simulink model "testBCIRobot3c"  (Simulink 10.0)
settings: Solver=FixedStepDiscrete  StartTime=0.0  StopTime=inf  FixedStep=0.002  MaxStep=0.02  RelTol=1e-3  AbsTol=1e-6
settings Model: Creator=fwornle  LastModifiedBy=bhisma  SimulationMode=external  ExtModeTrigDuration=5000  ExtModeLogAll=off
settings ConfigSet: Description=rtmc9s12target_R2009b
settings SolverCC: AutoScaleAbsTol=off
settings DataIOCC: SignalLoggingSaveFormat=ModelDataLogs  SaveOutput=off  SaveTime=off  SignalLoggingName=sigsOut
settings OptimizationCC: BlockReduction=off  BooleanDataType=off  ExpressionDepthLimit=2147483647  InitFltsAndDblsToZero=on  LifeSpan=1  EfficientTunableParamExpr=on
settings DebuggingCC: SaveWithParameterizedLinksMsg=none  SignalResolutionControl=TryResolveAllWithWarning  MultiTaskDSMMsg=warning  MultiTaskCondExecSysMsg=none  FcnCallInpInsideContextMsg=warning  StateNameClashWarn=warning
settings HardwareCC: ProdBitPerInt=16  ProdBitPerPointer=16  ProdBitPerSizeT=16  ProdBitPerPtrDiffT=16  ProdEndianess=BigEndian  ProdWordSize=16  ProdHWDeviceType=Motorola HC12
settings SFSimCC: MATLABDynamicMemAlloc=off
settings RTWCC: SystemTargetFile=mc9s12.tlc  GenerateMakefile=off  TemplateMakefile=mc9s12.tmf
settings CodeAppCC: IgnoreCustomStorageClasses=off  CustomSymbolStrType=$N$R$M  InternalIdentifier=Classic
settings STFCustomTargetCC: TargetFcnLib=ansi_tfl_tmw.mat  ModelReferenceCompliant=off  IncludeMdlTerminateFcn=off  ERTCustomFileBanners=on  SupportNonInlinedSFcns=off  RemoveResetFunc=on  MATLABClassNameForMDSCustomization=Simulink.SoftwareTarget.ERTCustomization  CPPClassGenCompliant=on  SystemTargetFile=mc9s12.tlc
settings ERTTargetCC: TargetFcnLib=ansi_tfl_tmw.mat  MultiwordLength=2048  ModelReferenceCompliant=off  ParMdlRefBuildCompliant=off  CompOptLevelCompliant=off  ConcurrentExecutionCompliant=off  IncludeMdlTerminateFcn=off  CombineOutputUpdateFcns=off  SupportContinuousTime=on  ModelStepFunctionPrototypeControlCompliant=off  GRTInterface=on  UseToolchainInfoCompliant=off  ExtMode=on  ExtModeMexFile=ext_serial_mc9s12_comm  ExtModeMexArgs=1,2,115200  ERTCustomFileTemplate=mc9s12_file_process.tlc  ConvertIfToSwitch=off  SuppressUnreachableDefaultCases=off
settings CustomProperty: DataType=RTWOptions_EnumType_C__Users_fw__SVN_rtmc9s12-target_trunk_rtmc9s12_CW_R2009b_bin_mc9s12_1mc9s12_TargetBoard  Value=MiniDragonPlus-RevE
settings EnumStrPairs: String=Dragon12
settings ConfigComp: CovExternalEMLEnable=off

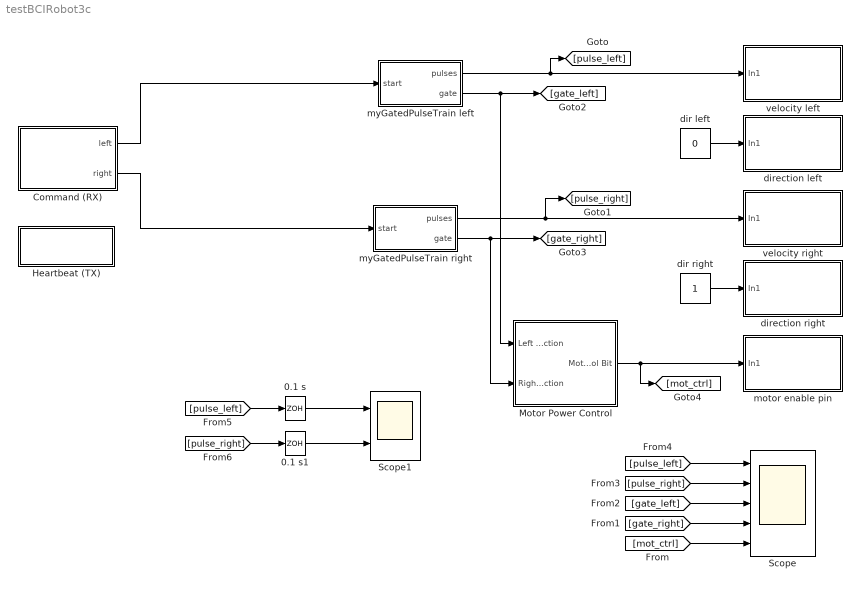
== system testBCIRobot3c ==
  0.1 s : ZeroOrderHold  SampleTime=0.1
  0.1 s1 : ZeroOrderHold  SampleTime=0.1
  Command (RX) : Subsystem
  Heartbeat (TX) : Subsystem  mask{Tbeat=3}
      mask prompts: Tbeat "Period of heartbeat signal (seconds)"
      mask Display: disp(['Tbeat = ' num2str(Tbeat) ' s'])
  Motor Power Control : Subsystem
  Scope : Scope  NumInputPorts=5
  Scope1 : Scope  NumInputPorts=2
  dir left : Constant  Value=0
  dir right : Constant
  direction left : Subsystem  Tag=mcTarget_digOut  mask{port=Port A, pin=5, sampletime=0.002, Von=0.5, Voff=0.5}
      mask prompts: port "Port (see hardware manuals for valid options)"; pin "Pin (see hardware manuals for valid options)"; sampletime "Sample time"; Von "On-threshold (Von)"; Voff "Off-threshold (Voff)"
      mask init:
      | [portstr, pinstr, pins] = mbc_digitaloutput(port, pin, sampletime, Von, Voff);
      mask Help: web('digOut_sfcn_9S12.html');
      mask TypeOptions port: Port A | Port B | Port H | Port J | Port M | Port P | Port S | Port T
      mask Display: fprintf('%s\nPins: %s', portstr, pinstr)
  direction right : Subsystem  Tag=mcTarget_digOut  mask{port=Port A, pin=7, sampletime=0.002, Von=0.5, Voff=0.5}
      mask prompts: port "Port (see hardware manuals for valid options)"; pin "Pin (see hardware manuals for valid options)"; sampletime "Sample time"; Von "On-threshold (Von)"; Voff "Off-threshold (Voff)"
      mask init:
      | [portstr, pinstr, pins] = mbc_digitaloutput(port, pin, sampletime, Von, Voff);
      mask Help: web('digOut_sfcn_9S12.html');
      mask TypeOptions port: Port A | Port B | Port H | Port J | Port M | Port P | Port S | Port T
      mask Display: fprintf('%s\nPins: %s', portstr, pinstr)
  motor enable pin : Subsystem  Tag=mcTarget_digOut  mask{port=Port T, pin=7, sampletime=0.002, Von=0.5, Voff=0.5}
      mask prompts: port "Port (see hardware manuals for valid options)"; pin "Pin (see hardware manuals for valid options)"; sampletime "Sample time"; Von "On-threshold (Von)"; Voff "Off-threshold (Voff)"
      mask init:
      | [portstr, pinstr, pins] = mbc_digitaloutput(port, pin, sampletime, Von, Voff);
      mask Help: web('digOut_sfcn_9S12.html');
      mask TypeOptions port: Port A | Port B | Port H | Port J | Port M | Port P | Port S | Port T
      mask Display: fprintf('%s\nPins: %s', portstr, pinstr)
  myGatedPulseTrain left : Subsystem  mask{Tcount=0.02, Nsamp=30}
      mask prompts: Tcount "Sample time"; Nsamp "Number of samples"
      mask init:
      | % each period has an on-phase and an off-phase
      | Ncount = 2*Nsamp;
  myGatedPulseTrain right : Subsystem  mask{Tcount=0.02, Nsamp=30}
      mask prompts: Tcount "Sample time"; Nsamp "Number of samples"
      mask init:
      | % each period has an on-phase and an off-phase
      | Ncount = 2*Nsamp;
  velocity left : Subsystem  Tag=mcTarget_digOut  mask{port=Port A, pin=4, sampletime=0.002, Von=0.5, Voff=0.5}
      mask prompts: port "Port (see hardware manuals for valid options)"; pin "Pin (see hardware manuals for valid options)"; sampletime "Sample time"; Von "On-threshold (Von)"; Voff "Off-threshold (Voff)"
      mask init:
      | [portstr, pinstr, pins] = mbc_digitaloutput(port, pin, sampletime, Von, Voff);
      mask Help: web('digOut_sfcn_9S12.html');
      mask TypeOptions port: Port A | Port B | Port H | Port J | Port M | Port P | Port S | Port T
      mask Display: fprintf('%s\nPins: %s', portstr, pinstr)
  velocity right : Subsystem  Tag=mcTarget_digOut  mask{port=Port A, pin=6, sampletime=0.002, Von=0.5, Voff=0.5}
      mask prompts: port "Port (see hardware manuals for valid options)"; pin "Pin (see hardware manuals for valid options)"; sampletime "Sample time"; Von "On-threshold (Von)"; Voff "Off-threshold (Voff)"
      mask init:
      | [portstr, pinstr, pins] = mbc_digitaloutput(port, pin, sampletime, Von, Voff);
      mask Help: web('digOut_sfcn_9S12.html');
      mask TypeOptions port: Port A | Port B | Port H | Port J | Port M | Port P | Port S | Port T
      mask Display: fprintf('%s\nPins: %s', portstr, pinstr)
  wires:
  Motor Power Control/1(Motor Control Bit) -> [mot_ctrl], motor enable pin/1(In1)
  myGatedPulseTrain left/2(gate) -> Motor Power Control/1(Left Motor Instruction), [gate_left]
  myGatedPulseTrain right/2(gate) -> Motor Power Control/2(Right Motor  Instruction), [gate_right]
  myGatedPulseTrain left/1(pulses) -> [pulse_left], velocity left/1(In1)
  myGatedPulseTrain right/1(pulses) -> [pulse_right], velocity right/1(In1)
  dir left/1 -> direction left/1(In1)
  dir right/1 -> direction right/1(In1)
  Command (RX)/2(right) -> myGatedPulseTrain right/1(start)
  [mot_ctrl] -> Scope/5
  [pulse_left] -> Scope/1
  [pulse_right] -> Scope/2
  [gate_left] -> Scope/3
  [gate_right] -> Scope/4
  Command (RX)/1(left) -> myGatedPulseTrain left/1(start)
  [pulse_left] -> 0.1 s/1
  [pulse_right] -> 0.1 s1/1
  0.1 s/1 -> Scope1/1
  0.1 s1/1 -> Scope1/2

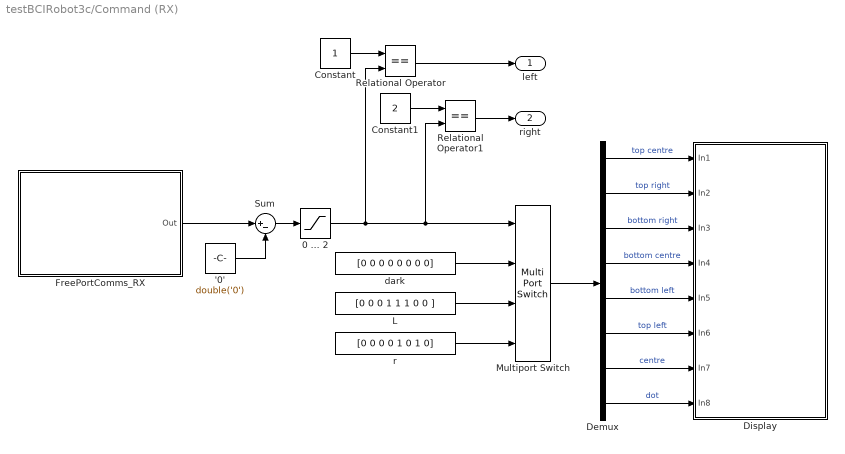
== system testBCIRobot3c/Command (RX) ==
  '0' : Constant  Value=double('0')
  0 ... 2 : Saturate  UpperLimit=2  LowerLimit=0
  Constant : Constant
  Constant1 : Constant  Value=2
  Demux : Demux  Outputs=8
  Display : Subsystem  Tag=mcTarget_digOut  mask{port=Port H, pin=0:7, sampletime=0.1, Von=0.5, Voff=0.5}
      mask prompts: port "Port (see hardware manuals for valid options)"; pin "Pin (see hardware manuals for valid options)"; sampletime "Sample time"; Von "On-threshold (Von)"; Voff "Off-threshold (Voff)"
      mask init:
      | [portstr, pinstr, pins] = mbc_digitaloutput(port, pin, sampletime, Von, Voff);
      mask Help: web('digOut_sfcn_9S12.html');
      mask TypeOptions port: Port A | Port B | Port H | Port J | Port M | Port P | Port S | Port T
      mask Display: fprintf('%s\nPins: %s', portstr, pinstr)
  FreePortComms_RX : Subsystem  Tag=mcTarget_freePortCommsRX  mask{sampletime=0.1, port=SCI0, baudrate=115200, channel=0, buf_size=1, data_type=UINT8, format=on, outformat=on}
      mask prompts: sampletime "Sample time"; port "Communication port"; channel "Channel number"; buf_size "Number of elements"; data_type "Data Type"; format "Block receives raw data"; outformat "Block output is double"
      mask init:
      | [buf_sizestr, portNamestr, baudratestr, channelstr, data_type_str, sampletime_str] = mbc_freeportrxd(sampletime, port, baudrate, channel, buf_size, data_type, format, outformat);
      mask Help: web('freePortComms_rxd.html');
      mask TypeOptions port: SCI0 | SCI1 | COM1 | COM2 | COM3 | COM4
      mask TypeOptions baudrate: 300 | 600 | 1200 | 2400 | 4800 | 9600 | 19200 | 38400 | 57600 | 115200
      mask TypeOptions data_type: SINGLE | INT8 | UINT8 | INT16 | UINT16 | INT32 | UINT32 | BOOLEAN
      mask Display: fprintf('Receive %s element(s)\nComm port: %s\nBaudrate: %s bps\nChannel: %s\nData type: %s\n Sample rate: %s', buf_sizestr, portNamestr, baudratestr, channelstr, data_type_str, sampletime_str)
  L : Constant  Value=[0 0 0 1 1 1 0 0 ]  OutDataTypeStr=double
  Multiport Switch : MultiPortSwitch  DataPortOrder=Zero-based contiguous  zeroidx=on  SaturateOnIntegerOverflow=on
  Relational Operator : RelationalOperator  Operator===  OutDataTypeStr=uint(8)  RndMeth=Nearest
  Relational Operator1 : RelationalOperator  Operator===  OutDataTypeStr=uint(8)  RndMeth=Nearest
  Sum : Sum  Inputs=|+-  SaturateOnIntegerOverflow=on
  dark : Constant  Value=[0 0 0 0 0 0 0 0]  OutDataTypeStr=double
  r : Constant  Value=[0 0 0 0 1 0 1 0]  OutDataTypeStr=double
  left : Outport
  right : Outport  Port=2
  wires:
  dark/1 -> Multiport Switch/2
  L/1 -> Multiport Switch/3
  r/1 -> Multiport Switch/4
  Constant/1 -> Relational Operator/1
  Relational Operator/1 -> left/1
  Constant1/1 -> Relational Operator1/1
  Relational Operator1/1 -> right/1
  Sum/1 -> 0 ... 2/1
  '0'/1 -> Sum/2
  FreePortComms_RX/1(Out) -> Sum/1
  Demux/1 -> Display/1(In1)  "top centre"
  Demux/2 -> Display/2(In2)  "top right"
  Demux/3 -> Display/3(In3)  "bottom right"
  Demux/4 -> Display/4(In4)  "bottom centre"
  Demux/5 -> Display/5(In5)  "bottom left"
  Demux/6 -> Display/6(In6)  "top left"
  Demux/7 -> Display/7(In7)  "centre"
  Demux/8 -> Display/8(In8)  "dot"
  Multiport Switch/1 -> Demux/1
  0 ... 2/1 -> Multiport Switch/1, Relational Operator1/2, Relational Operator/2

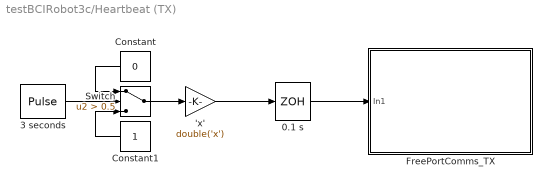
== system testBCIRobot3c/Heartbeat (TX) ==
  'x' : Gain  Gain=double('x')  SaturateOnIntegerOverflow=on  OutDataTypeStr=Inherit: Same as input  ParamDataTypeStr=Inherit: Same as input
  0.1 s : ZeroOrderHold  SampleTime=0.1
  3 seconds : DiscretePulseGenerator  PulseType=Time based  Period=3  PulseWidth=0.2
  Constant : Constant  Value=0
  Constant1 : Constant
  FreePortComms_TX : Subsystem  Tag=mcTarget_freePortCommsTX  mask{sampletime=0.1, port=SCI1, baudrate=115200, channel=0, buf_size=1, data_type=UINT8, format=on}
      mask prompts: sampletime "Sample time"; port "Communication port"; channel "Channel number"; buf_size "Number of elements"; data_type "Data Type"; format "Block sends raw data"
      mask init:
      | [buf_sizestr, portNamestr, baudratestr, channelstr, data_type_str, sampletime_str] = mbc_freeporttxd(sampletime, port, baudrate, channel, buf_size, data_type, format);
      mask Help: web('freePortComms_txd.html');
      mask TypeOptions port: SCI0 | SCI1 | COM1 | COM2 | COM3 | COM4
      mask TypeOptions baudrate: 300 | 600 | 1200 | 2400 | 4800 | 9600 | 19200 | 38400 | 57600 | 115200
      mask TypeOptions data_type: SINGLE | INT8 | UINT8 | INT16 | UINT16 | INT32 | UINT32 | BOOLEAN
      mask Display: fprintf('Transmit %s element(s)\nComm port: %s\nBaudrate: %s bps\nChannel: %s\nData type: %s\n Sample rate: %s', buf_sizestr, portNamestr, baudratestr, channelstr, data_type_str, sampletime_str)
  Switch : Switch  Criteria=u2 > Threshold  Threshold=0.5
  wires:
  0.1 s/1 -> FreePortComms_TX/1(In1)
  Constant/1 -> Switch/1
  3 seconds/1 -> Switch/2
  Constant1/1 -> Switch/3
  Switch/1 -> 'x'/1
  'x'/1 -> 0.1 s/1

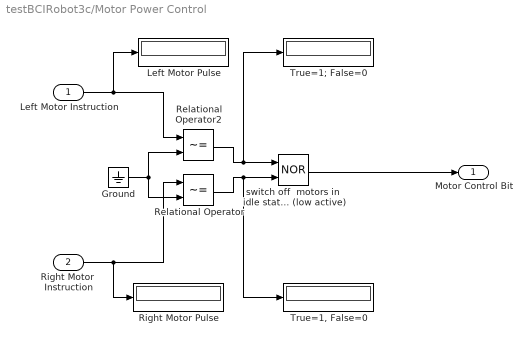
== system testBCIRobot3c/Motor Power Control ==
  Left Motor Instruction : Inport
  Right Motor  Instruction : Inport  Port=2
  Ground : Ground
  Left Motor Pulse : Display
  Relational Operator : RelationalOperator  Operator=~=  RndMeth=Nearest
  Relational Operator2 : RelationalOperator  Operator=~=  RndMeth=Nearest
  Right Motor Pulse : Display
  "True=1, False=0" : Display
  True=1; False=0 : Display
  switch off  motors in  idle state (low active) : Logic  Operator=NOR  AllPortsSameDT=off
  Motor Control Bit : Outport
  wires:
  Right Motor  Instruction/1 -> Relational Operator/1, Right Motor Pulse/1
  Left Motor Instruction/1 -> Relational Operator2/1, Left Motor Pulse/1
  Ground/1 -> Relational Operator2/2, Relational Operator/2
  Relational Operator2/1 -> switch off  motors in  idle state (low active)/1, True=1; False=0/1
  Relational Operator/1 -> switch off  motors in  idle state (low active)/2, "True=1, False=0"/1
  switch off  motors in  idle state (low active)/1 -> Motor Control Bit/1

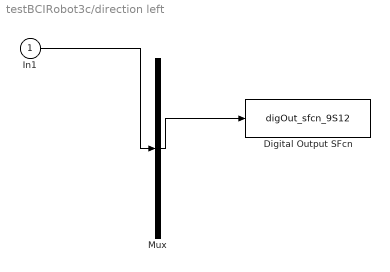
== system testBCIRobot3c/direction left ==
  In1 : Inport
  Digital Output SFcn : S-Function  Tag=mcTarget_digOut  FunctionName=digOut_sfcn_9S12  Parameters=sampletime, port, pins, Von, Voff  SFunctionDeploymentMode=off  EnableBusSupport=off
  Mux : Mux  Inputs=1
  wires:
  In1/1 -> Mux/1
  Mux/1 -> Digital Output SFcn/1

== system testBCIRobot3c/direction right ==
  In1 : Inport
  Digital Output SFcn : S-Function  Tag=mcTarget_digOut  FunctionName=digOut_sfcn_9S12  Parameters=sampletime, port, pins, Von, Voff  SFunctionDeploymentMode=off  EnableBusSupport=off
  Mux : Mux  Inputs=1
  wires:
  In1/1 -> Mux/1
  Mux/1 -> Digital Output SFcn/1

== system testBCIRobot3c/motor enable pin ==
  In1 : Inport
  Digital Output SFcn : S-Function  Tag=mcTarget_digOut  FunctionName=digOut_sfcn_9S12  Parameters=sampletime, port, pins, Von, Voff  SFunctionDeploymentMode=off  EnableBusSupport=off
  Mux : Mux  Inputs=1
  wires:
  In1/1 -> Mux/1
  Mux/1 -> Digital Output SFcn/1

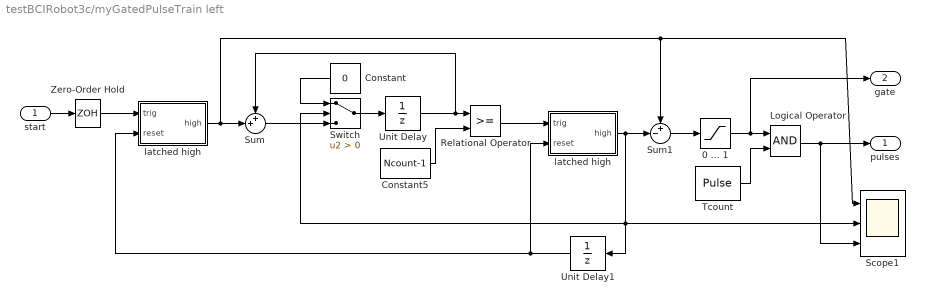
== system testBCIRobot3c/myGatedPulseTrain left ==
  start : Inport
  " latched high " : Subsystem
  0 ... 1 : Saturate  UpperLimit=1  LowerLimit=0
  Constant : Constant  Value=0
  Constant5 : Constant  Value=Ncount-1
  Logical Operator : Logic  AllPortsSameDT=off
  Relational Operator : RelationalOperator  OutDataTypeStr=uint(8)  RndMeth=Nearest
  Scope1 : Scope  NumInputPorts=3
  Sum : Sum  Inputs=++|
  Sum1 : Sum  Inputs=+-|
  Switch : Switch  Criteria=u2 > Threshold
  Tcount : DiscretePulseGenerator  SampleTime=Tcount
  Unit Delay : UnitDelay  SampleTime=Tcount
  Unit Delay1 : UnitDelay  SampleTime=Tcount
  Zero-Order Hold : ZeroOrderHold  SampleTime=Tcount
  latched high : Subsystem
  pulses : Outport
  gate : Outport  Port=2
  wires:
  Zero-Order Hold/1 -> latched high/1(trig)
  Logical Operator/1 -> Scope1/3, pulses/1
  Tcount/1 -> Logical Operator/2
  0 ... 1/1 -> gate/1, Logical Operator/1
  Unit Delay1/1 -> latched high/2(reset), " latched high "/2(reset)
  " latched high "/1(high) -> Unit Delay1/1, Switch/2, Scope1/2, Sum1/2
  Relational Operator/1 -> " latched high "/1(trig)
  Sum1/1 -> 0 ... 1/1
  Switch/1 -> Unit Delay/1
  Unit Delay/1 -> Sum/1, Relational Operator/1
  Sum/1 -> Switch/3
  Constant/1 -> Switch/1
  Constant5/1 -> Relational Operator/2
  start/1 -> Zero-Order Hold/1
  latched high/1(high) -> Scope1/1, Sum1/1, Sum/2

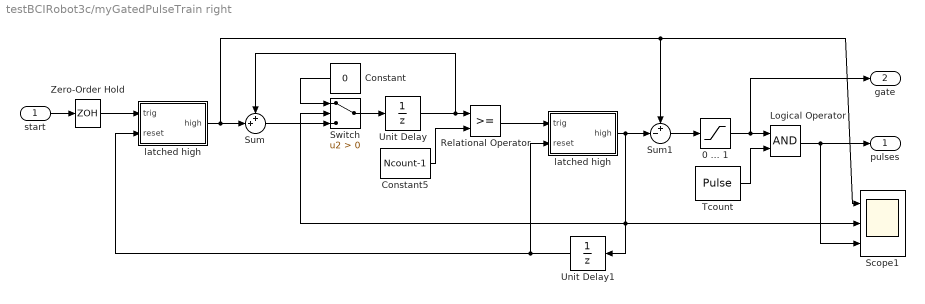
== system testBCIRobot3c/myGatedPulseTrain right ==
  start : Inport
  " latched high " : Subsystem
  0 ... 1 : Saturate  UpperLimit=1  LowerLimit=0
  Constant : Constant  Value=0
  Constant5 : Constant  Value=Ncount-1
  Logical Operator : Logic  AllPortsSameDT=off
  Relational Operator : RelationalOperator  OutDataTypeStr=uint(8)  RndMeth=Nearest
  Scope1 : Scope  NumInputPorts=3
  Sum : Sum  Inputs=++|
  Sum1 : Sum  Inputs=+-|
  Switch : Switch  Criteria=u2 > Threshold
  Tcount : DiscretePulseGenerator  SampleTime=Tcount
  Unit Delay : UnitDelay  SampleTime=Tcount
  Unit Delay1 : UnitDelay  SampleTime=Tcount
  Zero-Order Hold : ZeroOrderHold  SampleTime=Tcount
  latched high : Subsystem
  pulses : Outport
  gate : Outport  Port=2
  wires:
  latched high/1(high) -> Sum/2, Sum1/1, Scope1/1
  start/1 -> Zero-Order Hold/1
  Constant5/1 -> Relational Operator/2
  Constant/1 -> Switch/1
  Sum/1 -> Switch/3
  Unit Delay/1 -> Relational Operator/1, Sum/1
  Switch/1 -> Unit Delay/1
  Sum1/1 -> 0 ... 1/1
  Relational Operator/1 -> " latched high "/1(trig)
  " latched high "/1(high) -> Sum1/2, Scope1/2, Switch/2, Unit Delay1/1
  Unit Delay1/1 -> " latched high "/2(reset), latched high/2(reset)
  0 ... 1/1 -> Logical Operator/1, gate/1
  Tcount/1 -> Logical Operator/2
  Logical Operator/1 -> pulses/1, Scope1/3
  Zero-Order Hold/1 -> latched high/1(trig)

== system testBCIRobot3c/velocity left ==
  In1 : Inport
  Digital Output SFcn : S-Function  Tag=mcTarget_digOut  FunctionName=digOut_sfcn_9S12  Parameters=sampletime, port, pins, Von, Voff  SFunctionDeploymentMode=off  EnableBusSupport=off
  Mux : Mux  Inputs=1
  wires:
  Mux/1 -> Digital Output SFcn/1
  In1/1 -> Mux/1

== system testBCIRobot3c/velocity right ==
  In1 : Inport
  Digital Output SFcn : S-Function  Tag=mcTarget_digOut  FunctionName=digOut_sfcn_9S12  Parameters=sampletime, port, pins, Von, Voff  SFunctionDeploymentMode=off  EnableBusSupport=off
  Mux : Mux  Inputs=1
  wires:
  Mux/1 -> Digital Output SFcn/1
  In1/1 -> Mux/1

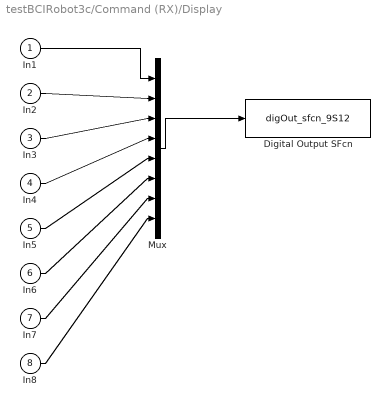
== system testBCIRobot3c/Command (RX)/Display ==
  In1 : Inport
  In2 : Inport  Port=2
  In3 : Inport  Port=3
  In4 : Inport  Port=4
  In5 : Inport  Port=5
  In6 : Inport  Port=6
  In7 : Inport  Port=7
  In8 : Inport  Port=8
  Digital Output SFcn : S-Function  Tag=mcTarget_digOut  FunctionName=digOut_sfcn_9S12  Parameters=sampletime, port, pins, Von, Voff  SFunctionDeploymentMode=off  EnableBusSupport=off
  Mux : Mux  Inputs=8
  wires:
  In1/1 -> Mux/1
  Mux/1 -> Digital Output SFcn/1
  In2/1 -> Mux/2
  In3/1 -> Mux/3
  In4/1 -> Mux/4
  In5/1 -> Mux/5
  In6/1 -> Mux/6
  In7/1 -> Mux/7
  In8/1 -> Mux/8

== system testBCIRobot3c/Command (RX)/FreePortComms_RX ==
  Data Type Conversion : DataTypeConversion  OutDataTypeStr=double  SaturateOnIntegerOverflow=on  RndMeth=Zero
  RECEIVE_FROM_FREE_PORT : S-Function  Tag=mcTarget_freePortCommsRX  FunctionName=freePortComms_rxd  Parameters=sampletime, channel, buf_size, data_type, port, baudrate, format  SFunctionDeploymentMode=off  EnableBusSupport=off
  Out : Outport
  wires:
  RECEIVE_FROM_FREE_PORT/1 -> Data Type Conversion/1
  Data Type Conversion/1 -> Out/1

== system testBCIRobot3c/Heartbeat (TX)/FreePortComms_TX ==
  In1 : Inport
  Data Type Conversion : DataTypeConversion  OutDataTypeStr=uint8  SaturateOnIntegerOverflow=on  RndMeth=Zero
  SEND_VIA_FREE_PORT : S-Function  Tag=mcTarget_freePortCommsTX  FunctionName=freePortComms_txd  Parameters=sampletime, channel, buf_size, data_type, port, baudrate, format  SFunctionDeploymentMode=off  EnableBusSupport=off
  wires:
  In1/1 -> Data Type Conversion/1
  Data Type Conversion/1 -> SEND_VIA_FREE_PORT/1

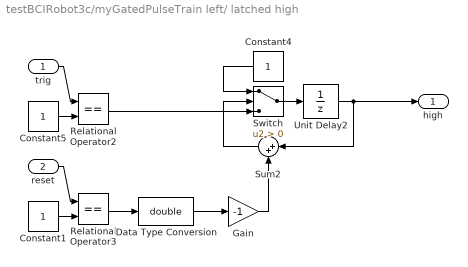
== system testBCIRobot3c/myGatedPulseTrain left/ latched high  ==
  trig : Inport
  reset : Inport  Port=2
  Constant1 : Constant
  Constant4 : Constant
  Constant5 : Constant
  Data Type Conversion : DataTypeConversion  OutDataTypeStr=double  SaturateOnIntegerOverflow=on  RndMeth=Zero
  Gain : Gain  Gain=-1  SaturateOnIntegerOverflow=on  OutDataTypeStr=Inherit: Same as input  ParamDataTypeStr=Inherit: Same as input
  Relational Operator2 : RelationalOperator  Operator===  OutDataTypeStr=uint(8)  RndMeth=Nearest
  Relational Operator3 : RelationalOperator  Operator===  OutDataTypeStr=uint(8)  RndMeth=Nearest
  Sum2 : Sum  Inputs=|++
  Switch : Switch  Criteria=u2 > Threshold
  Unit Delay2 : UnitDelay  SampleTime=-1
  high : Outport
  wires:
  trig/1 -> Relational Operator2/1
  reset/1 -> Relational Operator3/1
  Data Type Conversion/1 -> Gain/1
  Gain/1 -> Sum2/2
  Relational Operator3/1 -> Data Type Conversion/1
  Constant1/1 -> Relational Operator3/2
  Sum2/1 -> Switch/2
  Switch/1 -> Unit Delay2/1
  Constant4/1 -> Switch/1
  Unit Delay2/1 -> high/1, Sum2/1
  Relational Operator2/1 -> Switch/3
  Constant5/1 -> Relational Operator2/2

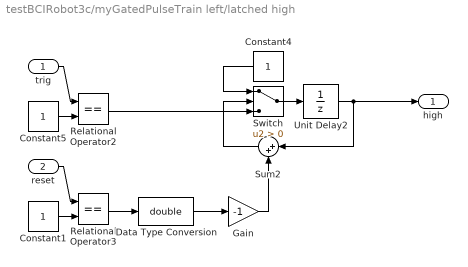
== system testBCIRobot3c/myGatedPulseTrain left/latched high ==
  trig : Inport
  reset : Inport  Port=2
  Constant1 : Constant
  Constant4 : Constant
  Constant5 : Constant
  Data Type Conversion : DataTypeConversion  OutDataTypeStr=double  SaturateOnIntegerOverflow=on  RndMeth=Zero
  Gain : Gain  Gain=-1  SaturateOnIntegerOverflow=on  OutDataTypeStr=Inherit: Same as input  ParamDataTypeStr=Inherit: Same as input
  Relational Operator2 : RelationalOperator  Operator===  OutDataTypeStr=uint(8)  RndMeth=Nearest
  Relational Operator3 : RelationalOperator  Operator===  OutDataTypeStr=uint(8)  RndMeth=Nearest
  Sum2 : Sum  Inputs=|++
  Switch : Switch  Criteria=u2 > Threshold
  Unit Delay2 : UnitDelay  SampleTime=-1
  high : Outport
  wires:
  Constant5/1 -> Relational Operator2/2
  Relational Operator2/1 -> Switch/3
  Unit Delay2/1 -> Sum2/1, high/1
  Constant4/1 -> Switch/1
  Switch/1 -> Unit Delay2/1
  Sum2/1 -> Switch/2
  Constant1/1 -> Relational Operator3/2
  Relational Operator3/1 -> Data Type Conversion/1
  Gain/1 -> Sum2/2
  Data Type Conversion/1 -> Gain/1
  reset/1 -> Relational Operator3/1
  trig/1 -> Relational Operator2/1

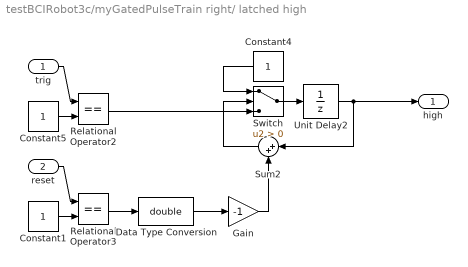
== system testBCIRobot3c/myGatedPulseTrain right/ latched high  ==
  trig : Inport
  reset : Inport  Port=2
  Constant1 : Constant
  Constant4 : Constant
  Constant5 : Constant
  Data Type Conversion : DataTypeConversion  OutDataTypeStr=double  SaturateOnIntegerOverflow=on  RndMeth=Zero
  Gain : Gain  Gain=-1  SaturateOnIntegerOverflow=on  OutDataTypeStr=Inherit: Same as input  ParamDataTypeStr=Inherit: Same as input
  Relational Operator2 : RelationalOperator  Operator===  OutDataTypeStr=uint(8)  RndMeth=Nearest
  Relational Operator3 : RelationalOperator  Operator===  OutDataTypeStr=uint(8)  RndMeth=Nearest
  Sum2 : Sum  Inputs=|++
  Switch : Switch  Criteria=u2 > Threshold
  Unit Delay2 : UnitDelay  SampleTime=-1
  high : Outport
  wires:
  Constant5/1 -> Relational Operator2/2
  Relational Operator2/1 -> Switch/3
  Unit Delay2/1 -> Sum2/1, high/1
  Constant4/1 -> Switch/1
  Switch/1 -> Unit Delay2/1
  Sum2/1 -> Switch/2
  Constant1/1 -> Relational Operator3/2
  Relational Operator3/1 -> Data Type Conversion/1
  Gain/1 -> Sum2/2
  Data Type Conversion/1 -> Gain/1
  reset/1 -> Relational Operator3/1
  trig/1 -> Relational Operator2/1

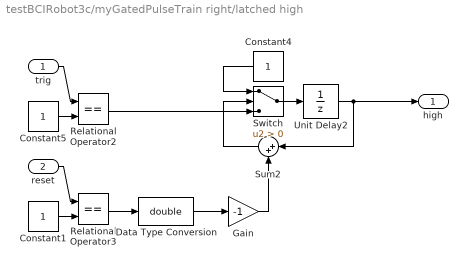
== system testBCIRobot3c/myGatedPulseTrain right/latched high ==
  trig : Inport
  reset : Inport  Port=2
  Constant1 : Constant
  Constant4 : Constant
  Constant5 : Constant
  Data Type Conversion : DataTypeConversion  OutDataTypeStr=double  SaturateOnIntegerOverflow=on  RndMeth=Zero
  Gain : Gain  Gain=-1  SaturateOnIntegerOverflow=on  OutDataTypeStr=Inherit: Same as input  ParamDataTypeStr=Inherit: Same as input
  Relational Operator2 : RelationalOperator  Operator===  OutDataTypeStr=uint(8)  RndMeth=Nearest
  Relational Operator3 : RelationalOperator  Operator===  OutDataTypeStr=uint(8)  RndMeth=Nearest
  Sum2 : Sum  Inputs=|++
  Switch : Switch  Criteria=u2 > Threshold
  Unit Delay2 : UnitDelay  SampleTime=-1
  high : Outport
  wires:
  trig/1 -> Relational Operator2/1
  reset/1 -> Relational Operator3/1
  Data Type Conversion/1 -> Gain/1
  Gain/1 -> Sum2/2
  Relational Operator3/1 -> Data Type Conversion/1
  Constant1/1 -> Relational Operator3/2
  Sum2/1 -> Switch/2
  Switch/1 -> Unit Delay2/1
  Constant4/1 -> Switch/1
  Unit Delay2/1 -> high/1, Sum2/1
  Relational Operator2/1 -> Switch/3
  Constant5/1 -> Relational Operator2/2
